simulink model "arduino_encoder1"  (R2023b)
settings: Solver=FixedStepAuto  StartTime=0.0  StopTime=inf  RelTol=1e-3  EnableMultiTasking=on
libraries: arduinolib x2
settings Model: ExtModeTrigDuration=2  Creator=yoany  LastModifiedBy=yoany
settings OptimizationCC: EnhancedBackFolding=on  PassReuseOutputArgsAs=Individual arguments  ZeroExternalMemoryAtStartup=off  ZeroInternalMemoryAtStartup=off  MaxStackSize=64  OptimizeBlockOrder=speed  DifferentSizesBufferReuse=on  OptimizationCustomize=off  EfficientTunableParamExpr=on
settings DebuggingCC: ParameterTunabilityLossMsg=error
settings HardwareCC: ProdBitPerPointer=32  ProdBitPerSizeT=32  ProdBitPerPtrDiffT=32  ProdLargestAtomicInteger=Long  ProdLargestAtomicFloat=Double  ProdWordSize=32  ProdHWDeviceType=ARM Compatible->ARM Cortex  UseEmbeddedCoderFeatures=off
settings SFSimCC: MATLABDynamicMemAlloc=off
settings RTWCC: Description=Embedded Coder  SystemTargetFile=ert.tlc  HardwareBoard=Arduino Nano 33 IoT  TemplateMakefile=ert_default_tmf  Toolchain=Arduino ARM  BuildConfiguration=Faster Runs
settings CodeAppCC: ForceParamTrailComments=on  IgnoreCustomStorageClasses=off  OperatorAnnotations=on  SimulinkDataObjDesc=on  SFDataObjDesc=on  InsertBlockDesc=on
settings ERTTargetCC: SupportContinuousTime=on  SupportNonInlinedSFcns=on  SupportVariableSizeSignals=on  ExtModeTransport=3  ExtModeStaticAlloc=on  ExtModeAutomaticAllocSize=off  ExtModeStaticAllocSize=8192  ExtModeMexFile=ext_xcp  ExtModeIntrfLevel=Level2 - Open

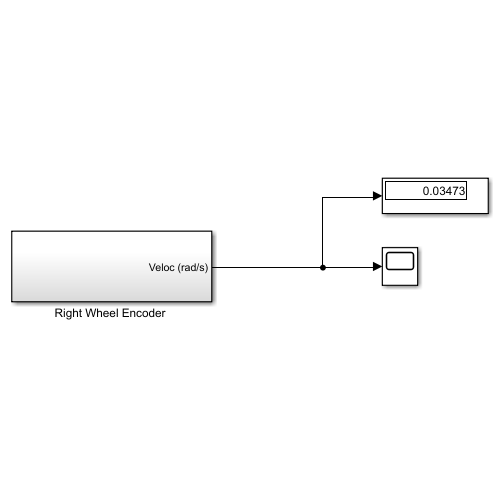
[thumbnail: Simulink's stored preview of the top-level diagram]
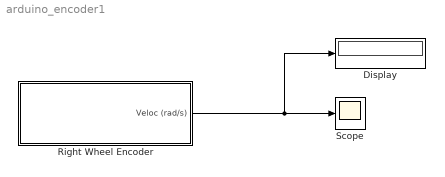
== system arduino_encoder1 ==
  Display : Display
  "Right Wheel Encoder " : Subsystem
  Scope : Scope
  wires:
  "Right Wheel Encoder "/1(Veloc (rad/s)) -> Display/1, Scope/1

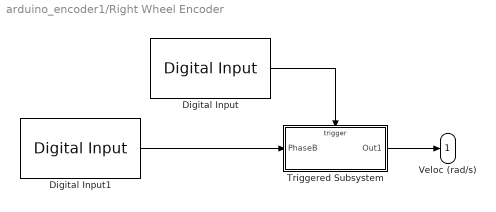
== system arduino_encoder1/Right Wheel Encoder  ==
  Digital Input : arduinolib/Digital Input  pinNumber=10  mode=Default  Direction=input  SampleTime=0.001  blockPlatform=arduino
  Digital Input1 : arduinolib/Digital Input  pinNumber=11  mode=Default  Direction=input  SampleTime=0.001  blockPlatform=arduino
  Triggered Subsystem : Subsystem  TreatAsAtomicUnit=on
  Veloc (rad/s) : Outport  VectorParamsAs1DForOutWhenUnconnected=off
  wires:
  Triggered Subsystem/1(Out1) -> Veloc (rad/s)/1
  Digital Input/1 -> Triggered Subsystem/Trigger
  Digital Input1/1 -> Triggered Subsystem/1(PhaseB)

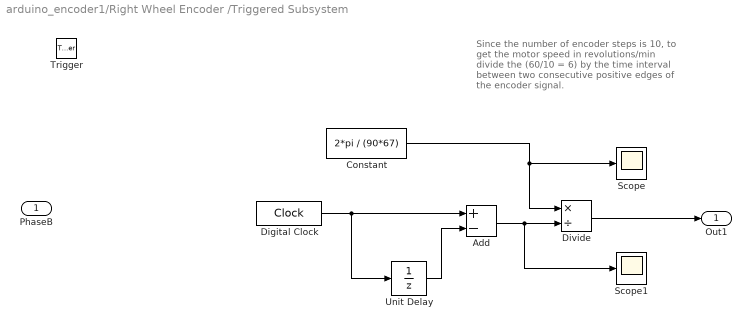
== system arduino_encoder1/Right Wheel Encoder /Triggered Subsystem ==
  note: Since the number of encoder steps is 10,
      | to get the motor speed in revolutions/min
      | divide the (60/10 = 6) by the time interval
      | between two consecutive positive edges
      | of the encoder signal.
  PhaseB : Inport
  Trigger : TriggerPort  VariantControl=Variant
  Add : Sum  Inputs=+-
  Constant : Constant  Value=2*pi / (90*67)
  Digital Clock : DigitalClock  SampleTime=-1
  Divide : Product  Inputs=*/
  Scope : Scope
  Scope1 : Scope
  Unit Delay : UnitDelay  SampleTime=-1  HasFrameUpgradeWarning=on
  Out1 : Outport  VectorParamsAs1DForOutWhenUnconnected=off
  wires:
  Digital Clock/1 -> Add/1, Unit Delay/1
  Unit Delay/1 -> Add/2
  Constant/1 -> Scope/1, Divide/1
  Add/1 -> Scope1/1, Divide/2
  Divide/1 -> Out1/1
